simulink model "OnlyDetectors"  (R2016b)
settings: Solver=FixedStepDiscrete  StartTime=0.0  StopTime=inf  FixedStep=sCoreParams.core.stepPeriod  RelTol=1e-3
undefined symbols (not defined in the file or in its folder): sCoreParams, sCoreParams_decoders_txDetector_detectChannelInds, sCoreParams_decoders_txDetector_txRMS, sCoreParams_decoders_txDetector_txSign
settings Model: DataTypeOverride=Double  MinMaxOverflowLogging=ForceOff  Creator=anish  LastModifiedBy=rzelmann
settings SolverCC: EnableConcurrentExecution=on
settings DataIOCC: SaveFormat=StructureWithTime  SignalLoggingSaveFormat=ModelDataLogs  SaveOutput=off  SignalLogging=off  DSMLogging=off  SaveTime=off
settings OptimizationCC: BlockReduction=off  BooleanDataType=off  ConditionallyExecuteInputs=off  DefaultParameterBehavior=Inlined  OptimizeBlockIOStorage=off  BufferReuse=off  GlobalBufferReuse=off  ExpressionFolding=off  LocalBlockOutputs=off  LifeSpan=inf
settings DebuggingCC: SignalRangeChecking=error  SaveWithParameterizedLinksMsg=none  SignalResolutionControl=TryResolveAllWithWarning  MultiTaskDSMMsg=warning  MultiTaskCondExecSysMsg=none  StateNameClashWarn=warning  SFUnexpectedBacktrackingDiag=warning  SFNoUnconditionalDefaultTransitionDiag=warning  SFExecutionAtInitializationDiag=none
settings HardwareCC: ProdBitPerPointer=32  ProdBitPerSizeT=32  ProdBitPerPtrDiffT=32  ProdLargestAtomicFloat=None  ProdWordSize=32  ProdLongLongMode=on  ProdHWDeviceType=Generic->32-bit x86 compatible  TargetBitPerPointer=64  TargetLargestAtomicFloat=Float  TargetLongLongMode=on  TargetIntDivRoundTo=Zero  TargetEndianess=LittleEndian  TargetWordSize=64  TargetHWDeviceType=Intel->x86-64 (Windows64)
settings ModelReferenceCC: UpdateModelReferenceTargets=Force  ModelReferenceNumInstancesAllowed=Single  ModelReferencePassRootInputsByReference=off
settings RTWCC: SystemTargetFile=slrt.tlc  TemplateMakefile=slrt_default_tmf  Description=Simulink Real-Time  BuildConfiguration=Faster Runs  RTWCompilerOptimization=on
settings ConfigComp: CovMetricSettings=dw  CovHtmlReporting=on  CovSaveCumulativeToWorkspaceVar=on  CovSaveSingleToWorkspaceVar=on  CovExternalEMLEnable=off  CovSFcnEnable=off

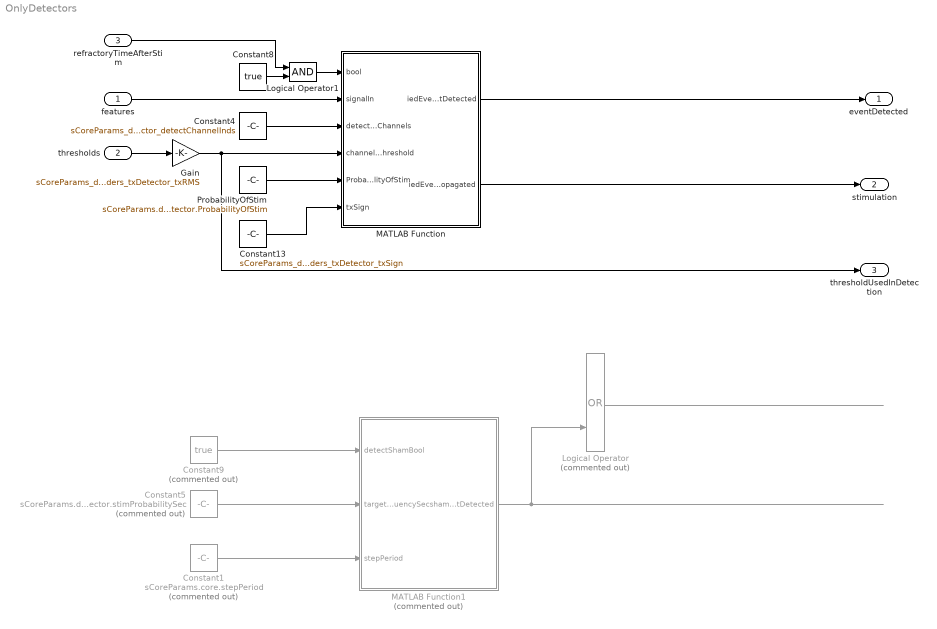
== system OnlyDetectors ==
  features : Inport  SampleTime=sCoreParams.core.stepPeriod
  thresholds : Inport  Port=2  SampleTime=sCoreParams.core.stepPeriod
  refractoryTimeAfterStim : Inport  Port=3  OutDataTypeStr=boolean  SampleTime=sCoreParams.core.stepPeriod
  Constant1 : Constant  Commented=on  Value=sCoreParams.core.stepPeriod
  Constant13 : Constant  Value=sCoreParams_decoders_txDetector_txSign
  Constant4 : Constant  Value=sCoreParams_decoders_txDetector_detectChannelInds
  Constant5 : Constant  Commented=on  Value=sCoreParams.decoders.chanceDetector.stimProbabilitySec
  Constant8 : Constant  Value=true
  Constant9 : Constant  Commented=on  Value=true
  Gain : Gain  Gain=sCoreParams_decoders_txDetector_txRMS
  Logical Operator : Logic  Commented=on  Operator=OR  AllPortsSameDT=off  OutDataTypeStr=boolean
  Logical Operator1 : Logic  IconShape=distinctive  AllPortsSameDT=off  OutDataTypeStr=boolean
  MATLAB Function : MATLAB Function  TreatAsAtomicUnit=on  SystemSampleTime=sCoreParams.core.stepPeriod
  MATLAB Function1 : MATLAB Function  Commented=on  TreatAsAtomicUnit=on  SystemSampleTime=sCoreParams.core.stepPeriod
  ProbabilityOfStim : Constant  Value=sCoreParams.decoders.txDetector.ProbabilityOfStim
  eventDetected : Outport  SampleTime=sCoreParams.core.stepPeriod
  stimulation : Outport  Port=2  SampleTime=sCoreParams.core.stepPeriod
  thresholdUsedInDetection : Outport  Port=3  SampleTime=sCoreParams.core.stepPeriod
  wires:
  Gain/1 -> MATLAB Function/4(channelThreshold), thresholdUsedInDetection/1
  MATLAB Function/2(iedEventPropagated) -> stimulation/1
  Constant4/1 -> MATLAB Function/3(detectableChannels)
  ProbabilityOfStim/1 -> MATLAB Function/5(ProbabilityOfStim)
  Logical Operator1/1 -> MATLAB Function/1(bool)
  Constant13/1 -> MATLAB Function/6(txSign)
  MATLAB Function/1(iedEventDetected) -> eventDetected/1
  features/1 -> MATLAB Function/2(signalIn)
  thresholds/1 -> Gain/1
  Constant1/1 -> MATLAB Function1/3(stepPeriod)
  Constant5/1 -> MATLAB Function1/2(targetShamFrequencySec)
  Constant9/1 -> MATLAB Function1/1(detectShamBool)
  MATLAB Function1/1(shamEventDetected) -> Logical Operator/2
  Logical Operator/1 -> ?
  refractoryTimeAfterStim/1 -> Logical Operator1/1
  Constant8/1 -> Logical Operator1/2

== matlab function OnlyDetectors/MATLAB Function1 ==
  data: detectShamBool input; shamEventDetected output; targetShamFrequencySec input; stepPeriod input
function shamEventDetected = ShamDetector(detectShamBool,targetShamFrequencySec,stepPeriod)
%#codegen

if detectShamBool
shamEventDetected = ShamDetector_EML(detectShamBool,targetShamFrequencySec,stepPeriod);
else
    shamEventDetected = false;
end

== matlab function OnlyDetectors/MATLAB Function ==
  data: bool input; iedEventDetected output boolean size=1; signalIn input; detectableChannels input; channelThreshold input; ProbabilityOfStim input; iedEventPropagated output boolean size=1; txSign input
function[iedEventDetected,iedEventPropagated] = InterictalTxDetector(bool,signalIn,detectableChannels,channelThreshold,ProbabilityOfStim,txSign)
%#codegen


[iedEventDetected,iedEventPropagated] = InterictalTxDetector_EML(bool,signalIn,detectableChannels,channelThreshold,ProbabilityOfStim);
%[iedEventDetected,iedEventPropagated] = TxPowerDetector_EML(bool, signalIn, detectableChannels, channelThreshold, shamProbability, txSign);
